simulink model "Gearbox_01test"  (Simulink 7.9)
settings: Solver=ode45  StartTime=0.0  StopTime=10.0  RelTol=1e-3
values from neighbouring files (symbols this model uses):
  Jc = 5.4e-5    (= 5.4e-05)    [Sim_Kinematik.m]    (also in Sim_Kinematik_mit_Getriebe.m)
undefined symbols (not defined in the file or in its folder): c_getr, d_getr, i_getr, M_last, Omega_in
settings Model: Creator=dep02378  LastModifiedBy=dep02378

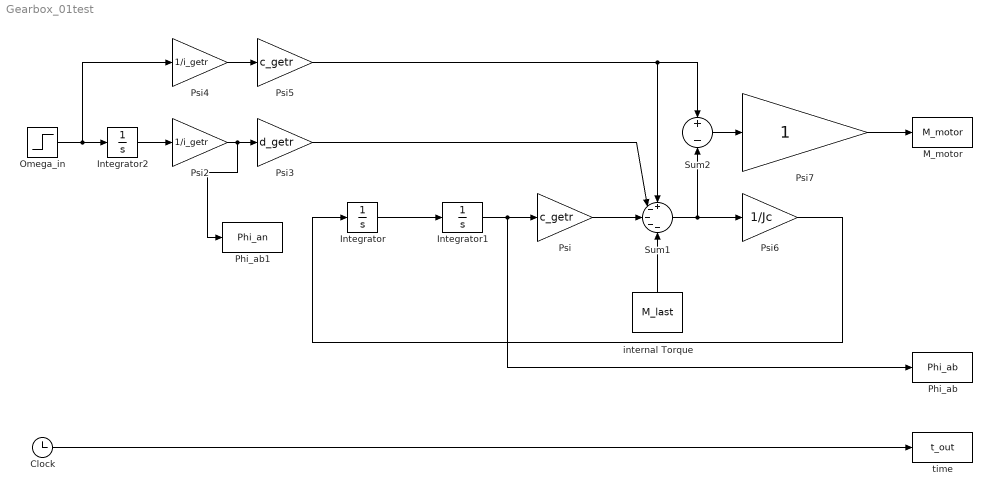
== system Gearbox_01test ==
  Clock : Clock
  Integrator : Integrator
  Integrator1 : Integrator
  Integrator2 : Integrator
  M_motor : ToWorkspace  VariableName=M_motor  SampleTime=-1
  Omega_in : Step  Time=0  After=Omega_in  SampleTime=0
  Phi_ab : ToWorkspace  VariableName=Phi_ab  SampleTime=-1
  Phi_ab1 : ToWorkspace  VariableName=Phi_an  SampleTime=-1
  Psi : Gain  Gain=c_getr
  Psi2 : Gain  Gain=1/i_getr
  Psi3 : Gain  Gain=d_getr
  Psi4 : Gain  Gain=1/i_getr
  Psi5 : Gain  Gain=c_getr
  Psi6 : Gain  Gain=1/Jc
  Psi7 : Gain
  Sum1 : Sum  Inputs=+----
  Sum2 : Sum  Inputs=+-
  internal Torque : Constant  Value=M_last
  time : ToWorkspace  VariableName=t_out  SampleTime=-1
  wires:
  Integrator/1 -> Integrator1/1
  Integrator1/1 -> Psi/1, Phi_ab/1
  Psi/1 -> Sum1/3
  Psi2/1 -> Psi3/1, Phi_ab1/1
  Psi4/1 -> Psi5/1
  Omega_in/1 -> Integrator2/1, Psi4/1
  Integrator2/1 -> Psi2/1
  Sum1/1 -> Psi6/1, Sum2/2
  Psi6/1 -> Integrator/1
  internal Torque/1 -> Sum1/5
  Psi5/1 -> Sum1/1, Sum2/1
  Sum2/1 -> Psi7/1
  Psi7/1 -> M_motor/1
  Clock/1 -> time/1
  Psi3/1 -> Sum1/2
